simulink model "try1"  (R2021b)
settings: Solver=VariableStepAuto  StartTime=0.0  StopTime=inf  RelTol=1e-3
libraries: sldrtlib x1
settings Model: Creator=danli  LastModifiedBy=danli

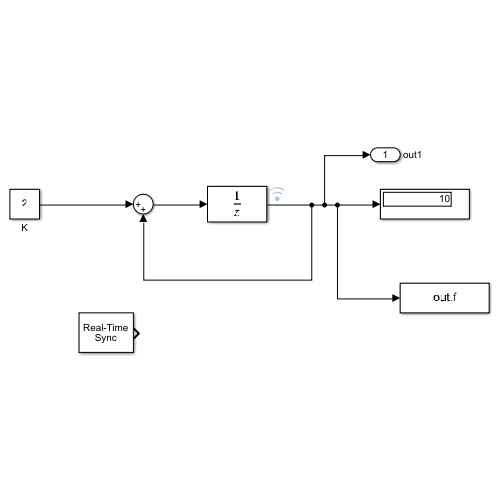
[thumbnail: Simulink's stored preview of the top-level diagram]
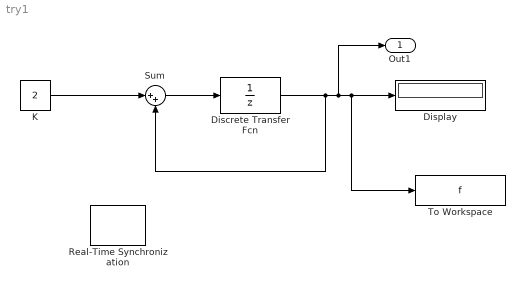
== system try1 ==
  Discrete Transfer Fcn : DiscreteTransferFcn  Denominator=[1 0]
  Display : Display
  K : Constant  Value=2
  Real-Time Synchronization : sldrtlib/Real-Time Synchronization  SampleTime=1  MaxMissedTicks=10  ShowMissedTicks=on  YieldWhenWaiting=off
  Sum : Sum  Inputs=|++
  To Workspace : ToWorkspace  VariableName=f  SampleTime=-1
      settings: Decimation=4  Save2DSignal=2-D array (concatenate along first dimension)
  Out1 : Outport  SignalName=out1
  wires:
  K/1 -> Sum/1
  Sum/1 -> Discrete Transfer Fcn/1
  Discrete Transfer Fcn/1 -> Sum/2, Out1/1, To Workspace/1, Display/1
